simulink model "chap02_03_49_mdl"  (R2013b)
settings: Solver=ode45  StartTime=0.0  StopTime=20  MaxStep=0.05  RelTol=1e-3
settings Model: Creator=Administrator  LastModifiedBy=sunzx.fnst

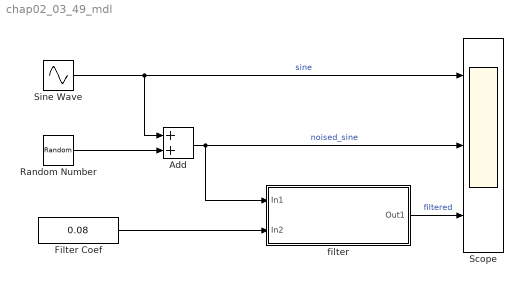
== system chap02_03_49_mdl ==
  Add : Sum
  Filter Coef : Constant  Value=0.08
      mask Display: fprintf('Filter coefficient');
  Random Number : RandomNumber  Variance=0.1
  Scope : Scope  NumInputPorts=3
      settings: YMin=-5~-5~-5  YMax=6~6~6
  Sine Wave : Sin  Amplitude=5  Frequency=0.5  SampleTime=0
  filter : Subsystem
      mask Display:
      | fprintf('filter');
      | port_label('input',1,'In1');
      | port_label('input',2,'In2');
      | port_label('output',1,'Out1');
  wires:
  filter/1(Out1) -> Scope/3  "filtered"
  Filter Coef/1 -> filter/2(In2)
  Add/1 -> Scope/2, filter/1(In1)  "noised_sine"
  Random Number/1 -> Add/2
  Sine Wave/1 -> Add/1, Scope/1  "sine"

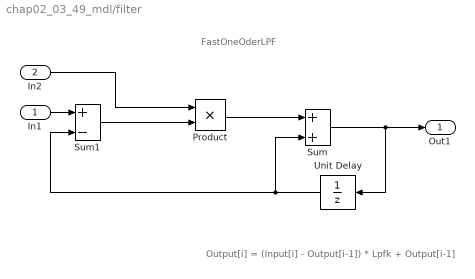
== system chap02_03_49_mdl/filter ==
  note: FastOneOderLPF
  note: Output[i] = (Input[i] - Output[i-1]) * Lpfk + Output[i-1]
  In1 : Inport
  In2 : Inport  Port=2
  Product : Product  RndMeth=Zero
  Sum : Sum
  Sum1 : Sum  Inputs=+-
  Unit Delay : UnitDelay  SampleTime=-1
  Out1 : Outport
  wires:
  Unit Delay/1 -> Sum/2, Sum1/2
  Product/1 -> Sum/1
  Sum/1 -> Unit Delay/1, Out1/1
  In1/1 -> Sum1/1
  Sum1/1 -> Product/2
  In2/1 -> Product/1
